simulink model "SSModel_r2018a"  (R2018a)
settings: Solver=VariableStepAuto  StartTime=0.0  StopTime=30  RelTol=1e-3
libraries: simulink x1
settings Model: Creator=SAI  LastModifiedBy=Arpit Mohakul
settings DebuggingCC: LibraryContextMissingDiagnostic=warning
settings SFSimCC: SimUseLocalCustomCode=on
settings RTWCC: RTWUseLocalCustomCode=on

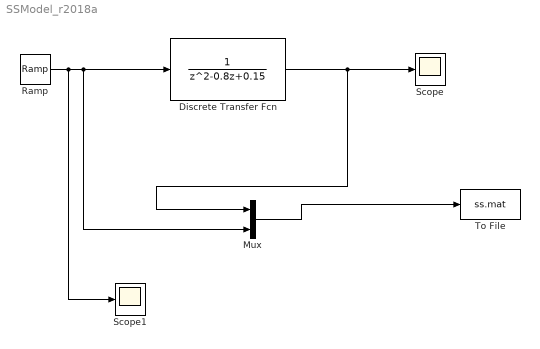
== system SSModel_r2018a ==
  Discrete Transfer Fcn : DiscreteTransferFcn  Numerator=[1]  Denominator=[1 -0.8 0.15]  SampleTime=0.1
  Mux : Mux  Inputs=2
  Ramp : simulink/Sources/Ramp  slope=3  start=0  InitialOutput=0
  Scope : Scope
  Scope1 : Scope
  To File : ToFile  Filename=ss.mat  MatrixName=a  SampleTime=0.1
  wires:
  Ramp/1 -> Scope1/1, Mux/2, Discrete Transfer Fcn/1
  Discrete Transfer Fcn/1 -> Mux/1, Scope/1
  Mux/1 -> To File/1
